simulink subsystem "Fault_Injector"  (R2023b)
settings: Solver=VariableStepAuto  StartTime=0.0  StopTime=10.0  RelTol=1e-3
libraries: simulink x8
settings Model: Creator=nickj  LastModifiedBy=diego

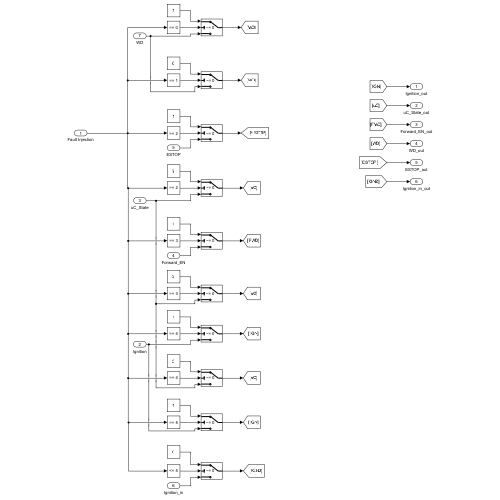
[thumbnail: Simulink's stored preview of the top-level diagram]
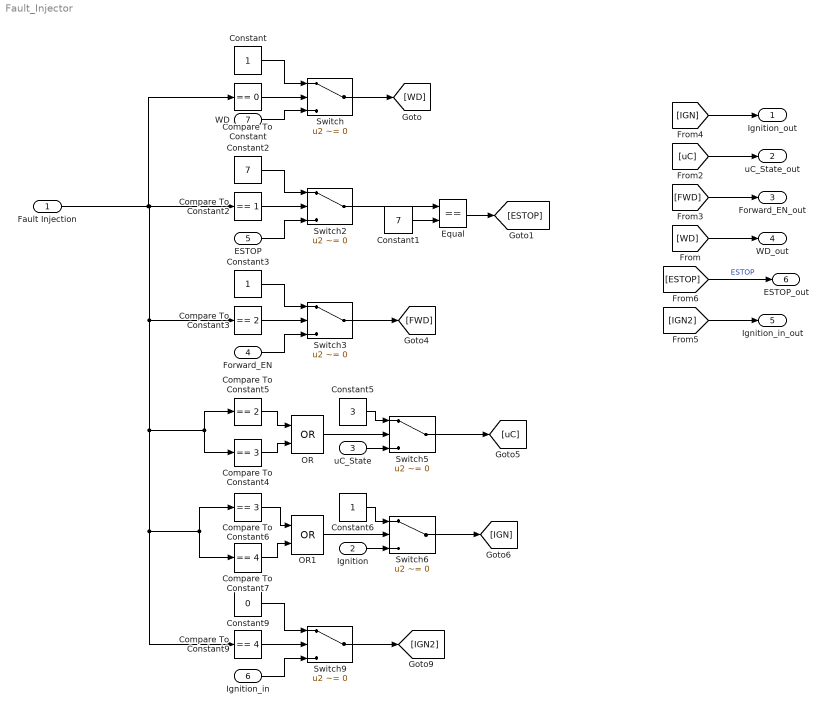
== system Fault_Injector ==
  Fault Injection : Inport
  Ignition : Inport  Port=2
  uC_State : Inport  Port=3
  Forward_EN : Inport  Port=4
  ESTOP : Inport  Port=5
  Ignition_in : Inport  Port=6
  WD : Inport  Port=7
  Compare To Constant : simulink/Logic and Bit Operations/Compare To Constant  relop===  const=0  OutDataTypeStr=boolean
  Compare To Constant2 : simulink/Logic and Bit Operations/Compare To Constant  relop===  const=1  OutDataTypeStr=boolean
  Compare To Constant3 : simulink/Logic and Bit Operations/Compare To Constant  relop===  const=2  OutDataTypeStr=boolean
  Compare To Constant4 : simulink/Logic and Bit Operations/Compare To Constant  relop===  const=3  OutDataTypeStr=boolean
  Compare To Constant5 : simulink/Logic and Bit Operations/Compare To Constant  relop===  const=2  OutDataTypeStr=boolean
  Compare To Constant6 : simulink/Logic and Bit Operations/Compare To Constant  relop===  const=3  OutDataTypeStr=boolean
  Compare To Constant7 : simulink/Logic and Bit Operations/Compare To Constant  relop===  const=4  OutDataTypeStr=boolean
  Compare To Constant9 : simulink/Logic and Bit Operations/Compare To Constant  relop===  const=4  OutDataTypeStr=boolean
  Constant : Constant
  Constant1 : Constant  Value=7
  Constant2 : Constant  Value=7
  Constant3 : Constant
  Constant5 : Constant  Value=3
  Constant6 : Constant
  Constant9 : Constant  Value=0
  Equal : RelationalOperator  Operator===  OutDataTypeStr=boolean  RndMeth=Simplest  InputSameDT=off
  OR : Logic  Operator=OR  IconShape=distinctive  AllPortsSameDT=off  OutDataTypeStr=boolean
  OR1 : Logic  Operator=OR  IconShape=distinctive  AllPortsSameDT=off  OutDataTypeStr=boolean
  Switch{,2..3,5..6,9} (6 alike) : Switch  Criteria=u2 ~= 0  SaturateOnIntegerOverflow=off  InputSameDT=off
  Ignition_out : Outport
  uC_State_out : Outport  Port=2
  Forward_EN_out : Outport  Port=3
  WD_out : Outport  Port=4
  Ignition_in_out : Outport  Port=5
  ESTOP_out : Outport  Port=6
  wires:
  Compare To Constant/1 -> Switch/2
  Constant/1 -> Switch/1
  Compare To Constant2/1 -> Switch2/2
  Constant2/1 -> Switch2/1
  Compare To Constant3/1 -> Switch3/2
  Constant3/1 -> Switch3/1
  Forward_EN/1 -> Switch3/3
  Switch/1 -> [WD]
  [WD] -> WD_out/1
  WD/1 -> Switch/3
  [uC] -> uC_State_out/1
  Switch3/1 -> [FWD]
  [FWD] -> Forward_EN_out/1
  Constant5/1 -> Switch5/1
  Switch5/1 -> [uC]
  Constant6/1 -> Switch6/1
  Ignition/1 -> Switch6/3
  Switch6/1 -> [IGN]
  [IGN] -> Ignition_out/1
  Ignition_in/1 -> Switch9/3
  Compare To Constant9/1 -> Switch9/2
  Constant9/1 -> Switch9/1
  Switch9/1 -> [IGN2]
  [IGN2] -> Ignition_in_out/1
  Compare To Constant5/1 -> OR/1
  OR/1 -> Switch5/2
  Compare To Constant4/1 -> OR/2
  uC_State/1 -> Switch5/3
  OR1/1 -> Switch6/2
  Compare To Constant6/1 -> OR1/1
  Compare To Constant7/1 -> OR1/2
  Fault Injection/1 -> Compare To Constant/1, Compare To Constant3/1, Compare To Constant4/1, Compare To Constant5/1, Compare To Constant7/1, Compare To Constant6/1, Compare To Constant9/1, Compare To Constant2/1
  ESTOP/1 -> Switch2/3
  [ESTOP] -> ESTOP_out/1  "ESTOP"
  Switch2/1 -> Equal/1
  Constant1/1 -> Equal/2
  Equal/1 -> [ESTOP]
